simulink model "final_arm_model"  (R2021b)
settings: Solver=VariableStepAuto  StartTime=0.0  StopTime=4.4  RelTol=1e-3
values from neighbouring files (symbols this model uses):
  AmpDen = [1 1.434e4 5.524e8]    [draft_model_variables.m]    (also in linear_model_variables.m)
  AmpNum = [1.393e9]    [draft_model_variables.m]    (also in linear_model_variables.m)
  CF = 1000    [derivative_filter.m]    (also in draft_model_variables.m = 1163; linear_model_variables.m = 1163)
  K1 = 60    [draft_model_variables.m]    (also in linear_model_variables.m = 50)
  K2 = 40    [draft_model_variables.m]    (also in linear_model_variables.m = 30)
  ka1 = km1    (= 0.0164)    [draft_model_variables.m]    (also in linear_model_variables.m)
  ka2 = km2    (= 0.0139)    [draft_model_variables.m]    (also in linear_model_variables.m)
  Kd1 = 0.03    [draft_model_variables.m]    (also in linear_model_variables.m = 0.00585120265616)
  Kd2 = 0.04    [draft_model_variables.m]    (also in linear_model_variables.m = 0.0123327238469)
  Ki1 = 0.7    [draft_model_variables.m]    (also in linear_model_variables.m = 1)
  Ki2 = 1.1    [draft_model_variables.m]    (also in linear_model_variables.m = 1)
  km1 = 16.4e-3    (= 0.0164)    [draft_model_variables.m]    (also in linear_model_variables.m)
  km2 = 13.9e-3    (= 0.0139)    [draft_model_variables.m]    (also in linear_model_variables.m)
  Kp1 = 0.3    [draft_model_variables.m]    (also in linear_model_variables.m = 0.153416231232)
  Kp2 = 0.22    [draft_model_variables.m]    (also in linear_model_variables.m = 0.222535517743)
  L1 = 0.245e-3    (= 0.000245)    [draft_model_variables.m]    (also in linear_model_variables.m)
  L2 = 0.0345e-3    (= 3.45e-05)    [draft_model_variables.m]    (also in linear_model_variables.m)
  N = 10    [derivative_filter.m]    (also in draft_model_variables.m = 100; linear_model_variables.m = 100)
  R1 = 0.115    [draft_model_variables.m]    (also in linear_model_variables.m)
  R2 = 0.2    [draft_model_variables.m]    (also in linear_model_variables.m)
  s = tf('s')    [draft_model_variables.m]    (also in linear_model_variables.m)
libraries: simulink x4, cstblocks x2
settings Model: Creator=ncamp  LastModifiedBy=ncamp

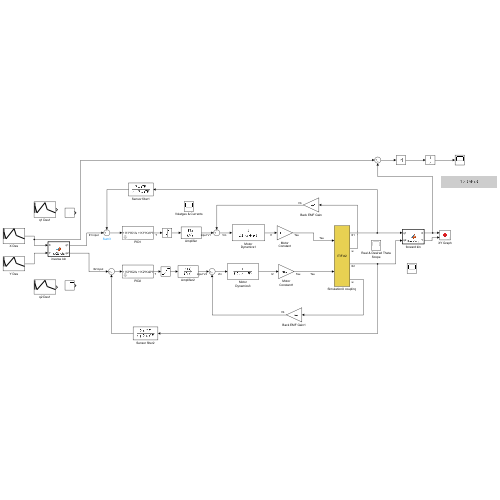
[thumbnail: Simulink's stored preview of the top-level diagram]
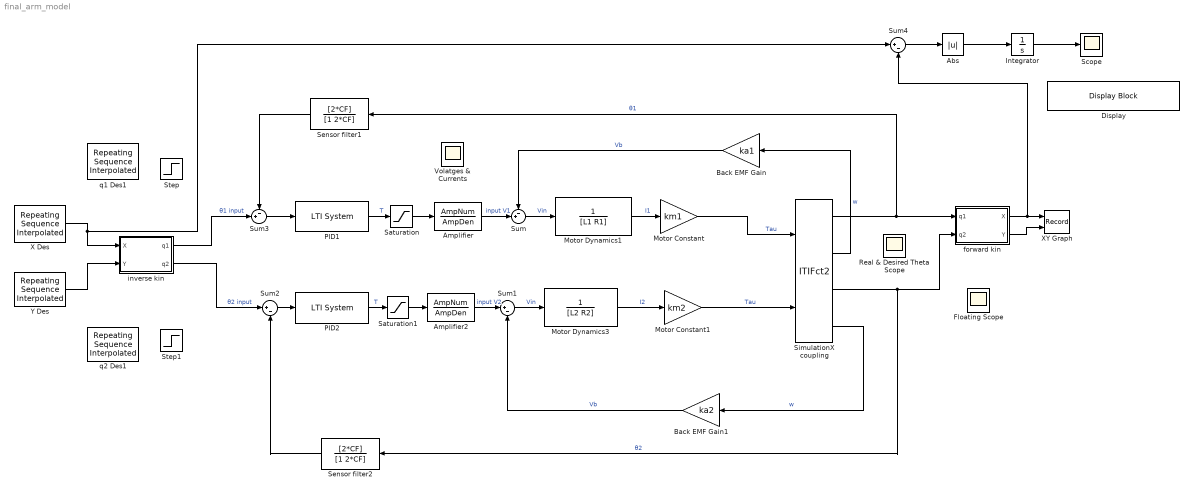
== system final_arm_model ==
  Abs : Abs
  Amplifier : TransferFcn  Numerator=AmpNum  Denominator=AmpDen
  Amplifier2 : TransferFcn  Numerator=AmpNum  Denominator=AmpDen
  Back EMF Gain : Gain  Gain=ka1
  Back EMF Gain1 : Gain  Gain=ka2
  Display : DisplayBlock  LabelPosition=Hide  Format=short  Transparency=1
  Floating Scope : Scope
      settings: Floating=on
  Integrator : Integrator
  Motor Constant : Gain  Gain=km1
  Motor Constant1 : Gain  Gain=km2
  Motor Dynamics1 : TransferFcn  Denominator=[L1 R1]
  Motor Dynamics3 : TransferFcn  Denominator=[L2 R2]
  PID1 : cstblocks/LTI System  sys=tf(K1*Kp1 + K1*Ki1/s + K1*Kd1*N*s/(s+N))  IC=[]
  PID2 : cstblocks/LTI System  sys=tf(K2*Kp2 + K2*Ki2/s + K2*Kd2*N*s/(s+N))  IC=[]
  Real & Desired Theta Scope : Scope
      settings: Floating=on
  Saturation : Saturate  UpperLimit=5  LowerLimit=-5
  Saturation1 : Saturate  UpperLimit=5  LowerLimit=-5
  Scope : Scope
  Sensor filter1 : TransferFcn  Numerator=[2*CF]  Denominator=[1 2*CF]
  Sensor filter2 : TransferFcn  Numerator=[2*CF]  Denominator=[1 2*CF]
  SimulationX coupling : S-Function  FunctionName=ITIFct2  Parameters=ip, port, ts, nIn, nOut  SFunctionDeploymentMode=off  EnableBusSupport=off  mask{ip='localhost', port=4097, ts=0.001, nIn=2, nOut=4}
      mask prompts: ip "Address: ip"; port "Port Number: port [-]"; ts "Communication Step Size: ts [s]"; nIn "Input Vector Dimension (to SimulationX): nIn [-]"; nOut "Output Vector Dimension (from SimulationX): nOut [-]"
      mask help: Coupling Element
  Step : Step  Time=0  After=0  SampleTime=0
  Step1 : Step  Time=0  After=pi/2  SampleTime=0
  Sum : Sum  Inputs=-+|
  Sum1 : Sum  Inputs=|+-
  Sum2 : Sum  Inputs=|+-
  Sum3 : Sum  Inputs=-+|
  Sum4 : Sum  Inputs=|+-
  Volatges & Currents : Scope
      settings: Floating=on
  X Des : simulink/Sources/Repeating Sequence Interpolated  OutValues=X  TimeValues=time  LookUpMeth=Interpolation-Use End Values  tsamp=0.001  OutMin=[]  OutMax=[]  OutDataTypeStr=double  OutputDataTypeScalingMode=double  OutDataType=fixdt(0,8)  OutScaling=2^-10
  XY Graph : Record  Filename=XYrecording.mldatx  RecordToWorkspace=on  FileSettingsInternal="{\"entries\":[{\"content\":{\"excelSettings\":{\"content\":{},\"type\":\"Streamout.ExcelSettings\"}},\"type\":\"Streamout.FileSettingStorage\",\"uuid\":\"80fa8e3e-65db-489b-9dbd-37fa92f46506\"}],\"packageUris\":[\"http://schema.mathworks.com/mf0/streamout_blocks/R2020a\"],\"version\":\"1.0\"}"  Layout=[1 2]  SignalsInternal="{\"entries\":[{\"content\":{\"signals\":[{\"content\":{\"blockPath\":[\"final_arm_model/XY Graph\"],\"channel\":[],\"dimensions\":[1],\"domain\":\"final_arm_model/XY Graph\",\"lineColor\":\"#a2142f\",\"plots\":[1],\"port\":1,\"sid\":[\"\"],\"signalID\":66016,\"signalName\":\"forward kin:1\"},\"type\":\"RecordBlkView.Signal\",\"uuid\":\"fe9b3bf2-487c-4c13-860b-649b138f007a\"},{\"content\":{\"blockPath\":[\"final_arm_model/XY Graph\"],\"channel\":[],\"dimensions\":[1],\"domain\":\"final_arm_model/XY Graph\",\"lineColor\":\"#139fff\",\"plots\":[1],\"port\":2,\"sid\":[\"\"],\"signalID\":66020,\"signalName\":\"forward kin:2\"},\"type\":\"RecordBlkView.Signal\",\"uuid\":\"644e1046-706f-43d6-b203-3565b06a1fca\"}]},\"type\":\"RecordBlkView.InputSignals\",\"uuid\":\"fd6f5bd4-ef38-4809-8d2f-17eece84b8fd\"}],\"packageUris\":[\"http://schema.mathworks.com/mf0/streamout_blocks/R2020a\"],\"version\":\"1.0\"}"  VisualizationBindings="{\"xyplotplugin\":{\"info\":[{\"series\":[{\"bindingParametersList\":[{\"parameter\":\"X-Axis\",\"signalID\":66016,\"signalName\":\"forward kin:1\"},{\"parameter\":\"Y-Axis\",\"signalID\":66020,\"signalName\":\"forward kin:2\"}],\"seriesID\":47805}],\"subplotID\":1}]}}"  CompatibilityTag=XY
  Y Des : simulink/Sources/Repeating Sequence Interpolated  OutValues=Y  TimeValues=time  LookUpMeth=Interpolation-Use End Values  tsamp=0.001  OutMin=[]  OutMax=[]  OutDataTypeStr=double  OutputDataTypeScalingMode=double  OutDataType=fixdt(0,8)  OutScaling=2^-10
  forward kin : MATLAB Function  TreatAsAtomicUnit=on
  inverse kin : MATLAB Function  TreatAsAtomicUnit=on
  q1 Des1 : simulink/Sources/Repeating Sequence Interpolated  OutValues=q1  TimeValues=time  LookUpMeth=Interpolation-Use End Values  tsamp=0.001  OutMin=[]  OutMax=[]  OutDataTypeStr=double  OutputDataTypeScalingMode=double  OutDataType=fixdt(0,8)  OutScaling=2^-10
  q2 Des1 : simulink/Sources/Repeating Sequence Interpolated  OutValues=q2  TimeValues=time  LookUpMeth=Interpolation-Use End Values  tsamp=0.001  OutMin=[]  OutMax=[]  OutDataTypeStr=double  OutputDataTypeScalingMode=double  OutDataType=fixdt(0,8)  OutScaling=2^-10
  wires:
  Back EMF Gain/1 -> Sum/1  "Vb"
  Motor Dynamics1/1 -> Motor Constant/1  "I1"
  Sum/1 -> Motor Dynamics1/1  "Vin"
  Back EMF Gain1/1 -> Sum1/2  "Vb"
  Motor Dynamics3/1 -> Motor Constant1/1  "I2"
  Sum1/1 -> Motor Dynamics3/1  "Vin"
  Sum2/1 -> PID2/1
  inverse kin/2(q2) -> Sum2/1  "θ2 input"
  PID2/1 -> Saturation1/1  "T"
  Amplifier2/1 -> Sum1/1  "input V2"
  PID1/1 -> Saturation/1  "T"
  Amplifier/1 -> Sum/2  "input V1"
  inverse kin/1(q1) -> Sum3/2  "θ1 input"
  Sum3/1 -> PID1/1
  Motor Constant1/1 -> SimulationX coupling/2  "Tau"
  Motor Constant/1 -> SimulationX coupling/1  "Tau"
  SimulationX coupling/2 -> Back EMF Gain/1  "w"
  SimulationX coupling/1 -> Sensor filter1/1, forward kin/1(q1)  "θ1"
  SimulationX coupling/4 -> Back EMF Gain1/1  "w"
  SimulationX coupling/3 -> forward kin/2(q2), Sensor filter2/1  "θ2"
  forward kin/1(X) -> Sum4/2, XY Graph/1
  forward kin/2(Y) -> XY Graph/2
  X Des/1 -> Sum4/1, inverse kin/1(X)
  Y Des/1 -> inverse kin/2(Y)
  Sensor filter2/1 -> Sum2/2
  Sensor filter1/1 -> Sum3/1
  Saturation/1 -> Amplifier/1
  Saturation1/1 -> Amplifier2/1
  Sum4/1 -> Abs/1
  Abs/1 -> Integrator/1
  Integrator/1 -> Scope/1

== matlab function final_arm_model/inverse kin ==
  data: X input; q1 output; Y input; q2 output
function [q1,q2] = xy2theta(X,Y)

% Inputs X,Y should be in mm
% Outputs q1, q2 are in rads

L1 = 275;   % Arm 1 length (mm)
L2 = 275;   % Arm 2 length (mm)

% Elbow down position
q1 = 2*atan((2*L1*Y - (- L1^4 + 2*L1^2*L2^2 + 2*L1^2*X^2 + 2*L1^2*Y^2 - L2^4 + 2*L2^2*X^2 + 2*L2^2*Y^2 - X^4 - 2*X^2*Y^2 - Y^4)^(1/2))/(L1^2 + 2*L1*X - L2^2 + X^2 + Y^2));
q2 =  2*atan(((- L1^2 + 2*L1*L2 - L2^2 + X^2 + Y^2)*(L1^2 + 2*L1*L2 + L2^2 - X^2 - Y^2))^(1/2)/(- L1^2 + 2*L1*L2 - L2^2 + X^2 + Y^2));


end

== matlab function final_arm_model/forward kin ==
  data: q1 input; X output; q2 input; Y output
function [X,Y] = theta2xy(q1,q2)

L1 = 275;
L2 = 275;

X = L1*cos(q1) + L2*cos(q1 + q2);
Y = L1*sin(q1) + L2*sin(q1 + q2);

end
